simulink model "cnn_accelerator"  (R2026a)
settings: Solver=VariableStepAuto
settings Model: Creator=svvb7  LastModifiedBy=svvb7

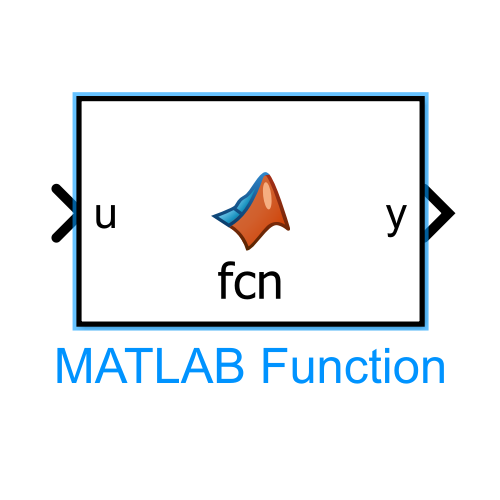
[thumbnail: Simulink's stored preview of the top-level diagram]
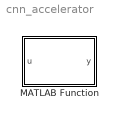
== system cnn_accelerator ==
  MATLAB Function : MATLAB Function  TreatAsAtomicUnit=on

== matlab function cnn_accelerator/MATLAB Function ==
  data: u input; y output
function y = fcn(u)
clc;
clear;
close all;

model = 'cnn_accelerator';

new_system(model);

open_system(model);

% Input
add_block('simulink/Sources/In1', ...
    [model '/Image_Input']);

% Convolution
add_block('simulink/Math Operations/Product', ...
    [model '/Convolution']);

% ReLU
add_block('simulink/Math Operations/Abs', ...
    [model '/ReLU']);

% Pooling
add_block('simulink/Math Operations/MinMax', ...
    [model '/MaxPooling']);

% Output
add_block('simulink/Sinks/Out1', ...
    [model '/CNN_Output']);

% Connections
add_line(model,'Image_Input/1','Convolution/1');

add_line(model,'Convolution/1','ReLU/1');

add_line(model,'ReLU/1','MaxPooling/1');

add_line(model,'MaxPooling/1','CNN_Output/1');

save_system(model);

open_system(model);
